simulink model "SMIB_start"  (Simulink 7.2)
settings: Solver=ode3  SolverMode=SingleTasking  StartTime=0.0  StopTime=15  FixedStep=1e-4  RelTol=1e-3
values from neighbouring files (symbols this model uses):
  D = 0.01    [MODEL_WORKSPACE.mat]    (also in MODEL_WORKSPACE_53.mat; WS.mat)
  J = 20    [MODEL_WORKSPACE.mat]    (also in MODEL_WORKSPACE_53.mat; WS.mat)
  Rf = 0.00246    [MODEL_WORKSPACE.mat]    (also in MODEL_WORKSPACE_53.mat = 0.0025; WS.mat = 0.0025)
  Tdo = 3    [MODEL_WORKSPACE.mat]    (also in MODEL_WORKSPACE_53.mat; WS.mat)
  Vbus = 1    [MODEL_WORKSPACE.mat]    (also in MODEL_WORKSPACE_53.mat; WS.mat)
  X = 0.4    [MODEL_WORKSPACE.mat]    (also in MODEL_WORKSPACE_53.mat; WS.mat)
  Xd = 1    [MODEL_WORKSPACE.mat]    (also in MODEL_WORKSPACE_53.mat; WS.mat)
  Xdp = 0.25    [MODEL_WORKSPACE.mat]    (also in MODEL_WORKSPACE_53.mat; WS.mat)
  Xf = 0.8    [MODEL_WORKSPACE.mat]    (also in MODEL_WORKSPACE_53.mat; WS.mat)
libraries: simulink x2, powerlib x1
settings Model: Creator=F  LastModifiedBy=F
settings OptimizationCC: BlockReduction=off  BooleanDataType=off  ExpressionDepthLimit=128
settings DebuggingCC: SaveWithParameterizedLinksMsg=none  SignalResolutionControl=TryResolveAllWithWarning  SolverPrmCheckMsg=none  FcnCallInpInsideContextMsg=Enable All  StateNameClashWarn=none  StrictBusMsg=ErrorLevel1
settings HardwareCC: TargetUnknown=on
settings CodeAppCC: CustomSymbolStrType=$N$R$M_T
settings GRTTargetCC: TargetFunctionLibrary=C89/C90 (ANSI)

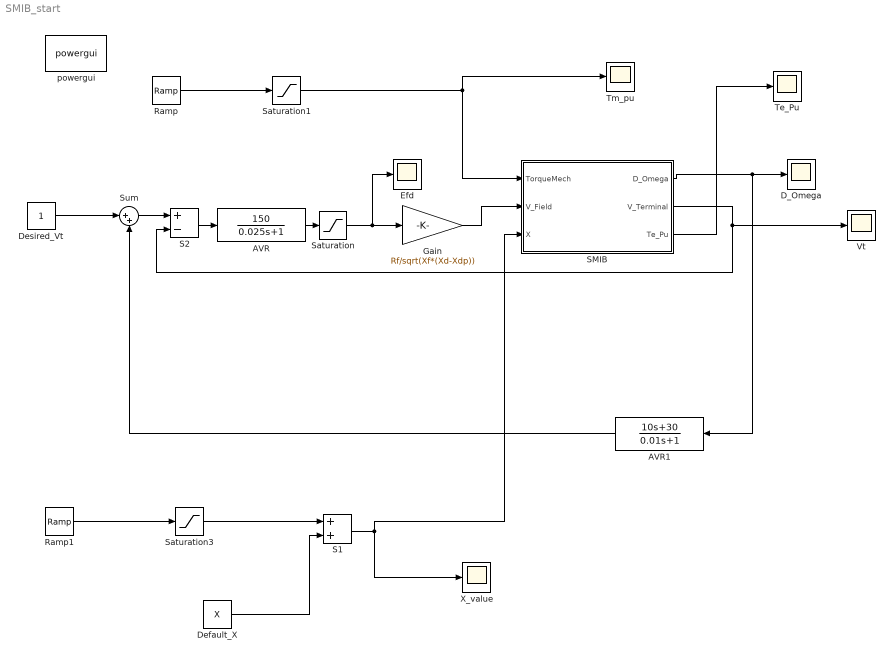
== system SMIB_start ==
  AVR : TransferFcn  Numerator=[150]  Denominator=[0.025 1]
  AVR1 : TransferFcn  Orientation=left  Numerator=[10 30]  Denominator=[0.01 1]
  D_Omega : Scope
      settings: YMin=-0.01  YMax=0.0125  DataFormat=Array  MaxDataPoints=500000
  Default_X : Constant  Value=X
  Desired_Vt : Constant
  Efd : Scope
      settings: YMin=0  YMax=2  DataFormat=Array  MaxDataPoints=500000
  Gain : Gain  Gain=Rf/sqrt(Xf*(Xd-Xdp))
  Ramp : simulink/Sources/Ramp  SystemSampleTime=-1  slope=0.3  start=0  X0=0
  Ramp1 : simulink/Sources/Ramp  SystemSampleTime=-1  slope=-100000  start=0.8  X0=10000
  S1 : Sum
  S2 : Sum  Inputs=+-
  SMIB : Subsystem
  Saturation : Saturate  UpperLimit=1.9  LowerLimit=0
  Saturation1 : Saturate  UpperLimit=1  LowerLimit=0
  Saturation3 : Saturate  UpperLimit=X*1000  LowerLimit=0
  Sum : Sum  Inputs=|++
  Te_Pu : Scope
      settings: YMin=0  YMax=2.25  DataFormat=Array  MaxDataPoints=500000
  Tm_pu : Scope
      settings: YMin=0  YMax=0.525  DataFormat=Array  MaxDataPoints=500000
  Vt : Scope
      settings: TimeRange=30  YMin=0  YMax=1.1  DataFormat=Array  MaxDataPoints=500000
  X_value : Scope
      settings: YMin=0  YMax=4.5  SaveName=ScopeData2  DataFormat=Array  MaxDataPoints=500000
  powergui : powerlib/powergui  Priority=1  SystemSampleTime=-1  SimulationMode=Continuous  SampleTime=50e-6  frequency=60  SPID=off  DisableSnubberDevices=off  DisableRonSwitches=off  DisableVfSwitches=off  SwTol=0  Interpol=off  frequencyindice=60  echomessages=off  HookPort=off  FunctionMessages=off  EnableUseOfTLC=off  x0status=blocks  RestoreLinks=warning  Frange=[0:2:500]  Ylog=off  Xlog=on  ShowGrid=off  save=off  variable=ZData  structure=0  ZoomFFT=off  StartTime=0.0  cycles=1  DisplayStyle=1  fundamental=60  FreqAxis=off  MaxFrequency=1000  frequencyindicesteady=1  RmsSteady=1  display=off  Ts=0  methode=off
  wires:
  S2/1 -> AVR/1
  SMIB/2(V_Terminal) -> S2/2, Vt/1
  SMIB/3(Te_Pu) -> Te_Pu/1
  Gain/1 -> SMIB/2(V_Field)
  Sum/1 -> S2/1
  Desired_Vt/1 -> Sum/1
  SMIB/1(D_Omega) -> D_Omega/1, AVR1/1
  AVR/1 -> Saturation/1
  Saturation/1 -> Efd/1, Gain/1
  Ramp/1 -> Saturation1/1
  Saturation1/1 -> SMIB/1(TorqueMech), Tm_pu/1
  S1/1 -> SMIB/3(X), X_value/1
  Ramp1/1 -> Saturation3/1
  Saturation3/1 -> S1/1
  Default_X/1 -> S1/2
  AVR1/1 -> Sum/2

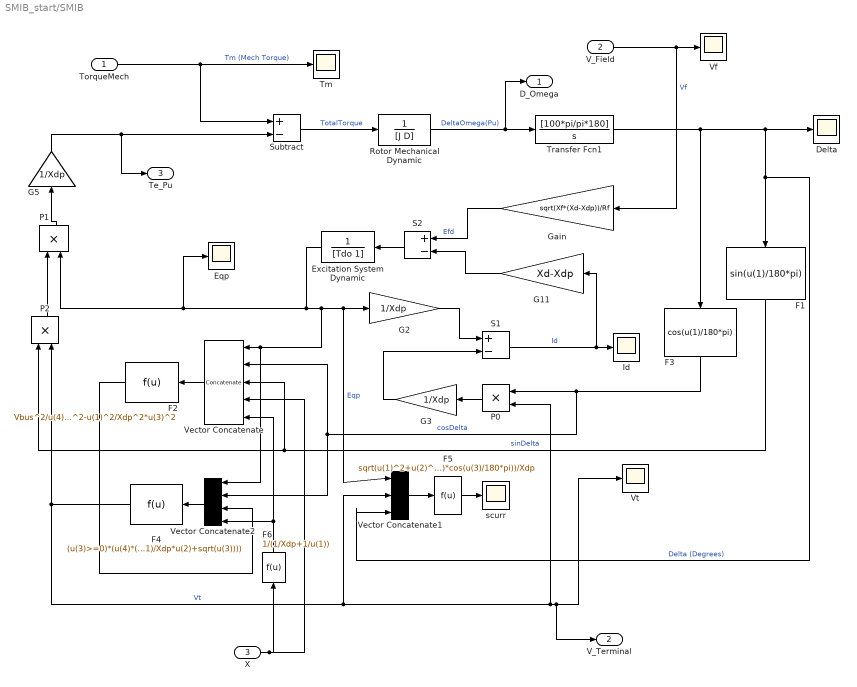
== system SMIB_start/SMIB ==
  TorqueMech : Inport
  V_Field : Inport  Port=2
  X : Inport  Port=3
  Delta : Scope
      settings: YMin=-10  YMax=60  DataFormat=Array  MaxDataPoints=500000
  Eqp : Scope
      settings: DataFormat=Array
  Excitation System Dynamic : TransferFcn  Orientation=left  Denominator=[Tdo 1]
  F1 : Fcn  Orientation=down  Expr=sin(u(1)/180*pi)
  F2 : Fcn  Orientation=left  Expr=Vbus^2/u(4)^2-u(1)^2/Xdp^2*u(3)^2
  F3 : Fcn  Orientation=down  Expr=cos(u(1)/180*pi)
  F4 : Fcn  Orientation=left  Expr=(u(3)>=0)*(u(4)*(u(1)/Xdp*u(2)+sqrt(u(3))))
  F5 : Fcn  Expr=sqrt(u(1)^2+u(2)^2-2*u(1)*u(2)*cos(u(3)/180*pi))/Xdp
  F6 : Fcn  Orientation=up  Expr=1/(1/Xdp+1/u(1))
  G11 : Gain  Orientation=left  Gain=Xd-Xdp
  G2 : Gain  Gain=1/Xdp
  G3 : Gain  Orientation=left  Gain=1/Xdp
  G5 : Gain  Orientation=up  Gain=1/Xdp
  Gain : Gain  Orientation=left  Gain=sqrt(Xf*(Xd-Xdp))/Rf
  Id : Scope
      settings: DataFormat=Array
  P0 : Product  Orientation=left
  P1 : Product  Orientation=up
  P2 : Product  Orientation=up
  Rotor Mechanical Dynamic : TransferFcn  Denominator=[J D]
  S1 : Sum  Inputs=+-
  S2 : Sum  Orientation=left  Inputs=+-
  Subtract : Sum  Inputs=+-
  Tm : Scope
      settings: DataFormat=Array
  Transfer Fcn1 : TransferFcn  Numerator=[100*pi/pi*180]  Denominator=[1 0]
  Vector Concatenate : Concatenate  Orientation=left  NumInputs=5  Mode=Vector
  Vector Concatenate1 : Concatenate  NumInputs=3  Mode=Vector
  Vector Concatenate2 : Concatenate  Orientation=left  NumInputs=4  Mode=Vector
  Vf : Scope
      settings: DataFormat=Array
  Vt : Scope
      settings: DataFormat=Array
  scurr : Scope
      settings: YMin=0  YMax=2.75  SaveName=ScopeData3  DataFormat=Array  MaxDataPoints=500000
  D_Omega : Outport
  V_Terminal : Outport  Port=2
  Te_Pu : Outport  Port=3
  wires:
  Rotor Mechanical Dynamic/1 -> D_Omega/1, Transfer Fcn1/1  "DeltaOmega(Pu)"
  Subtract/1 -> Rotor Mechanical Dynamic/1  "TotalTorque"
  S2/1 -> Excitation System Dynamic/1
  Gain/1 -> S2/1  "Efd"
  G11/1 -> S2/2
  Excitation System Dynamic/1 -> Vector Concatenate/1, Vector Concatenate2/1, G2/1, Vector Concatenate1/1, Eqp/1, P1/2  "Eqp"
  V_Field/1 -> Vf/1, Gain/1  "Vf"
  S1/1 -> Id/1, G11/1  "Id"
  G2/1 -> S1/1
  G3/1 -> S1/2
  P0/1 -> G3/1
  P1/1 -> G5/1
  F1/1 -> Vector Concatenate/3, P2/1  "sinDelta"
  TorqueMech/1 -> Tm/1, Subtract/1  "Tm (Mech Torque)"
  F3/1 -> P0/1, Vector Concatenate/2, Vector Concatenate2/2  "cosDelta"
  Transfer Fcn1/1 -> Delta/1, F1/1, Vector Concatenate1/3, F3/1  "Delta (Degrees)"
  F4/1 -> P2/2, P0/2, V_Terminal/1, Vt/1, Vector Concatenate1/2  "Vt"
  Vector Concatenate/1 -> F2/1
  X/1 -> Vector Concatenate/4, F6/1
  G5/1 -> Subtract/2, Te_Pu/1
  P2/1 -> P1/1
  F6/1 -> Vector Concatenate/5, Vector Concatenate2/4
  F2/1 -> Vector Concatenate2/3
  Vector Concatenate2/1 -> F4/1
  F5/1 -> scurr/1
  Vector Concatenate1/1 -> F5/1
